simulink model "modules"  (R2017a)
settings: Solver=ode4  StartTime=0.0  StopTime=time_stop  FixedStep=time_step  RelTol=1e-3
values from neighbouring files (symbols this model uses):
  psi = state(3)    [PSVobstacleShip_class.m]    (also in PSVvessel_class.m = obj.eta(3); PsiReferenceModel_class.m = obj.desired_psi_vector; SBMPC_PSVvessel_class.m = obj.eta(3))
undefined symbols (not defined in the file or in its folder): beta, Delta_guidance, Delta_matrix, eta_initial, initial_desired_psi_vector, initial_desired_u_vector, initial_next_waypoint_indexes, initial_obstacle_ship_states, initial_obstacle_ship_states_dot, initial_reference_psi_vector, initial_reference_u_vector, initial_SBMPC_desired_psi_vector, initial_SBMPC_desired_u_vector, initial_SBMPC_next_waypoint_indexes, initial_SBMPC_obstacle_ship_states, initial_SBMPC_obstacle_ship_states_dot, initial_SBMPC_reference_psi_vector, initial_SBMPC_reference_u_vector, initial_SBMPC_x_d_psi_matrix, initial_SBMPC_x_d_u_matrix, initial_state, initial_x_d_psi_matrix, initial_x_d_u_matrix, K_sway, K_yaw, Kp_feedback_linearization, kp_heading, Nmax, nu_initial, num_obs_ship_waypoints, num_prediction_time_steps, number_of_control_behaviors, number_of_obstacle_ships, number_of_SBMPC_obstacle_ships, obs_speed_between_waypoints, obstacle_waypoint_matrix, Omega_matrix, own_ship_reference_psi_init, own_ship_reference_speed, Psi_init, radius_of_acceptance, SBMPC_obs_speed_between_waypoints, SBMPC_obstacle_waypoint_matrix, seconds_between_prediction, state_vector_init, T, T_k_surge, T_k_sway, T_k_yaw, T_s, T_waypoints, time_step, tsamp, U, U_init, V_init, waypoints_obstacle_ships, waypoints_own_ship, Xmax, Ymax
(part 1 of 5)
settings Model: TunableVars=eta_initial,nu_initial,waypoints_own_ship,waypoints_own_ship_straight_path  TunableVarsStorageClass=Auto,Auto,Auto,Auto  TunableVarsTypeQualifier=,,,  Creator=krikjers  LastModifiedBy=Kristian
settings DataIOCC: SaveFormat=Structure
settings RTWCC: SystemTargetFile=grtfmi.tlc  GenerateMakefile=off  TemplateMakefile=none  Description=FMU based on GRT (Functional Mock-up Unit)  RetainRTWFile=on
settings STFCustomTargetCC: TargetLangStandard=C99 (ISO)  CombineOutputUpdateFcns=on  MultiInstanceERTCode=on  CodeInterfacePackaging=Reusable function  GRTInterface=off  GenerateAllocFcn=on  SystemTargetFile=grtfmi.tlc
settings GRTTargetCC: ParMdlRefBuildCompliant=off  CompOptLevelCompliant=off  ConcurrentExecutionCompliant=off  MatFileLogging=off  MultiInstanceERTCode=on  CodeInterfacePackaging=Reusable function  CPPClassGenCompliant=off  GenerateAllocFcn=on  UseToolchainInfoCompliant=off

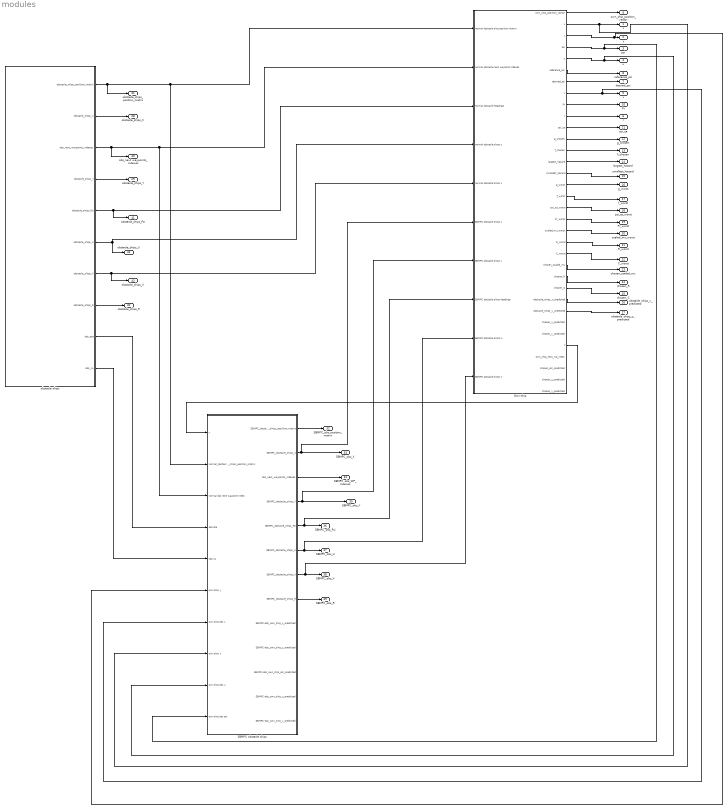
== system modules ==
  Own-ship : Subsystem
  SBMPC obstacle ships : Subsystem
  obstacle ships : Subsystem
  x : Outport
  y : Outport  Port=2
  psi : Outport  Port=3
  u : Outport  Port=4
  v : Outport  Port=5
  r : Outport  Port=6
  desired_psi : Outport  Port=7
  reference_psi : Outport  Port=8
  "own_ship_position_vector " : Outport  Port=9
  Pr : Outport  Port=10
  "psi_ca " : Outport  Port=11
  "g_chosen " : Outport  Port=12  SampleTime=time_step
  f_chosen : Outport  Port=13  SampleTime=time_step
  largest_hazard : Outport  Port=14  SampleTime=time_step
  smallest_hazard : Outport  Port=15  SampleTime=time_step
  "g_worst " : Outport  Port=16  SampleTime=time_step
  f_worst : Outport  Port=17  SampleTime=time_step
  psi_ca_worst : Outport  Port=18  SampleTime=time_step
  Pr_worst : Outport  Port=19  SampleTime=time_step
  scaled_mu_worst : Outport  Port=20  SampleTime=time_step
  R_worst : Outport  Port=21  SampleTime=time_step
  C_worst : Outport  Port=22  SampleTime=time_step
  chosen_scaled_mu : Outport  Port=23  SampleTime=time_step
  chosen_R : Outport  Port=24  SampleTime=time_step
  chosen_C : Outport  Port=25  SampleTime=time_step
  obstacle_ships_x_predicted : Outport  Port=26  SampleTime=time_step
  "obstacle_ships_y_predicted " : Outport  Port=27  SampleTime=time_step
  obstacle_ships_X : Outport  Port=28
  obstacle_ships_Y : Outport  Port=29
  obstacle_ships_R : Outport  Port=30
  "obstacle_ships_position_matrix " : Outport  Port=31
  "SBMPC_obs_position_matrix " : Outport  Port=32
  SBMPC_obs_X : Outport  Port=33
  SBMPC_obs_WP_indexes : Outport  Port=34
  SBMPC_obs_Y : Outport  Port=35
  SBMPC_obs_Psi : Outport  Port=36
  SBMPC_obs_U : Outport  Port=37
  SBMPC_obs_V : Outport  Port=38
  SBMPC_obs_R : Outport  Port=39
  obs_next_waypoints_indexes : Outport  Port=40
  obstacle_ships_Psi : Outport  Port=41
  obstacle_ships_U : Outport  Port=42
  obstacle_ships_V : Outport  Port=43
  wires:
  obstacle ships/2(obstacle_ships_X) -> obstacle_ships_X/1
  obstacle ships/4(obstacle_ships_Y) -> obstacle_ships_Y/1
  obstacle ships/5(obstacle_ships_Psi) -> obstacle_ships_Psi/1, Own-ship/3(normal obstacle headings)
  obstacle ships/6(obstacle_ships_U) -> obstacle_ships_U/1, Own-ship/4(normal obstacle ships u)
  obstacle ships/7(obstacle_ships_V) -> obstacle_ships_V/1, Own-ship/5(normal obstacle ships v)
  obstacle ships/8(obstacle_ships_R) -> obstacle_ships_R/1
  obstacle ships/3(obs_next_waypoints_indexes) -> obs_next_waypoints_indexes/1, Own-ship/2(normal obstacle next waypoint indexes), SBMPC obstacle ships/3(normal obs next waypoint index)
  Own-ship/1("own_ship_position_vector ") -> "own_ship_position_vector "/1
  Own-ship/2(x) -> SBMPC obstacle ships/8("own ship  x "), x/1
  Own-ship/6(reference_psi) -> reference_psi/1
  Own-ship/7(desired_psi) -> desired_psi/1
  Own-ship/9(Pr) -> Pr/1
  Own-ship/10(r) -> r/1
  Own-ship/11("psi_ca ") -> "psi_ca "/1
  Own-ship/12("g_chosen ") -> "g_chosen "/1
  Own-ship/13(f_chosen) -> f_chosen/1
  Own-ship/14(largest_hazard) -> largest_hazard/1
  Own-ship/15(smallest_hazard) -> smallest_hazard/1
  Own-ship/16("g_worst ") -> "g_worst "/1
  Own-ship/17(f_worst) -> f_worst/1
  Own-ship/18(psi_ca_worst) -> psi_ca_worst/1
  Own-ship/19(Pr_worst) -> Pr_worst/1
  Own-ship/20(scaled_mu_worst) -> scaled_mu_worst/1
  Own-ship/21(R_worst) -> R_worst/1
  Own-ship/22(C_worst) -> C_worst/1
  Own-ship/23(chosen_scaled_mu) -> chosen_scaled_mu/1
  Own-ship/24(chosen_R) -> chosen_R/1
  Own-ship/25(chosen_C) -> chosen_C/1
  Own-ship/26(obstacle_ships_x_predicted) -> obstacle_ships_x_predicted/1
  Own-ship/27("obstacle_ships_y_predicted ") -> "obstacle_ships_y_predicted "/1
  SBMPC obstacle ships/7(SBMPC_obstacle_ships_V) -> SBMPC_obs_V/1, Own-ship/10("SBMPC obstacle ships V ")
  SBMPC obstacle ships/6(SBMPC_obstacle_ships_U) -> Own-ship/9("SBMPC obstacle ships U "), SBMPC_obs_U/1
  SBMPC obstacle ships/5(SBMPC_obstacle_ships_Psi) -> Own-ship/8("SBMPC obstacle ships headings "), SBMPC_obs_Psi/1
  SBMPC obstacle ships/8(SBMPC_obstacle_ships_R) -> SBMPC_obs_R/1
  SBMPC obstacle ships/4(SBMPC_obstacle_ships_Y) -> Own-ship/7("SBMPC obstacle ships y "), SBMPC_obs_Y/1
  SBMPC obstacle ships/3(obs_next_waypoints_indexes) -> SBMPC_obs_WP_indexes/1
  SBMPC obstacle ships/2(SBMPC_obstacle_ships_X) -> Own-ship/6("SBMPC obstacle ships x "), SBMPC_obs_X/1
  SBMPC obstacle ships/1("SBMPC_obstacle_ships_positiion_matrix ") -> "SBMPC_obs_position_matrix "/1
  Own-ship/30(t) -> SBMPC obstacle ships/1(t)
  obstacle ships/9(obs_eta) -> SBMPC obstacle ships/4(obs eta)
  obstacle ships/10(obs_nu) -> SBMPC obstacle ships/5(obs nu)
  obstacle ships/1("obstacle_ships_positiion_matrix ") -> "obstacle_ships_position_matrix "/1, SBMPC obstacle ships/2(normal_obstacle_ships_position_matrix), Own-ship/1("normal obstacle ship position matrix ")
  Own-ship/5(u) -> SBMPC obstacle ships/9("own ship obs u "), u/1
  Own-ship/8(v) -> SBMPC obstacle ships/7("own ship obs v "), v/1
  Own-ship/4(psi) -> SBMPC obstacle ships/10("own ship obs psi "), psi/1
  Own-ship/3(y) -> SBMPC obstacle ships/6("own ship  y "), y/1

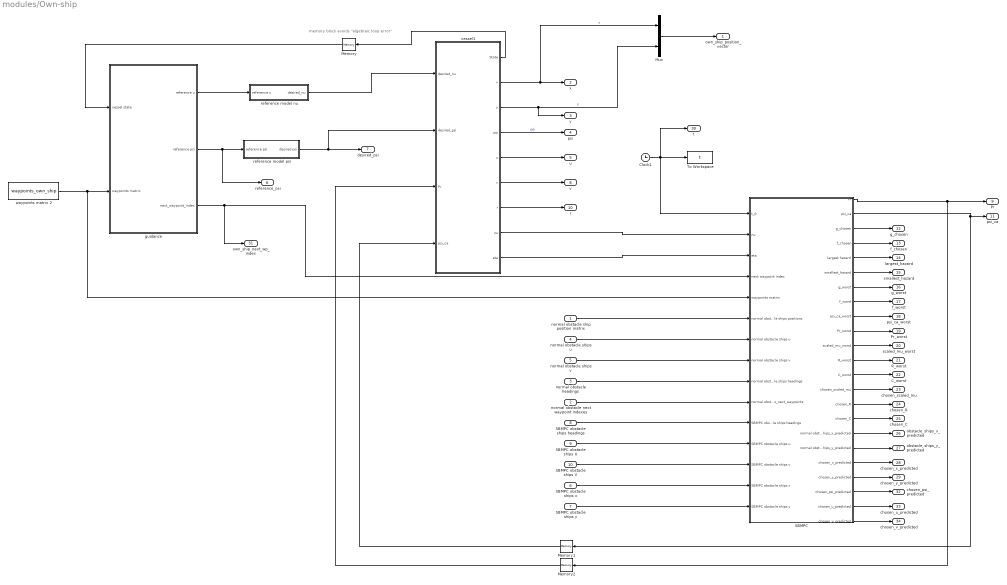
== system modules/Own-ship ==
  note: memory block avoids "algebraic loop error"
  "normal obstacle ship position matrix " : Inport
  normal obstacle next waypoint indexes : Inport  Port=2
  normal obstacle headings : Inport  Port=3
  normal obstacle ships u : Inport  Port=4
  normal obstacle ships v : Inport  Port=5
  "SBMPC obstacle ships x " : Inport  Port=6
  "SBMPC obstacle ships y " : Inport  Port=7
  "SBMPC obstacle ships headings " : Inport  Port=8
  "SBMPC obstacle ships U " : Inport  Port=9
  "SBMPC obstacle ships V " : Inport  Port=10
  Clock1 : Clock
  Memory : Memory  X0=initial_state  InheritSampleTime=on
  Memory1 : Memory  InheritSampleTime=on
  Memory2 : Memory  InheritSampleTime=on
  Mux : Mux  Inputs=2
  "SBMPC " : Subsystem
  To Workspace : ToWorkspace  VariableName=t  SampleTime=tsamp
  guidance : Subsystem
  reference model nu : Subsystem
  reference model psi : Subsystem
  vessel1 : Subsystem
  waypoints matrix 2 : Constant  Value=waypoints_own_ship  VectorParams1D=off  SampleTime=time_step
  "own_ship_position_vector " : Outport
  x : Outport  Port=2
  y : Outport  Port=3
  psi : Outport  Port=4
  u : Outport  Port=5
  reference_psi : Outport  Port=6
  desired_psi : Outport  Port=7
  v : Outport  Port=8
  Pr : Outport  Port=9
  r : Outport  Port=10
  "psi_ca " : Outport  Port=11
  "g_chosen " : Outport  Port=12  SampleTime=time_step
  f_chosen : Outport  Port=13  SampleTime=time_step
  largest_hazard : Outport  Port=14  SampleTime=time_step
  smallest_hazard : Outport  Port=15  SampleTime=time_step
  "g_worst " : Outport  Port=16  SampleTime=time_step
  f_worst : Outport  Port=17  SampleTime=time_step
  psi_ca_worst : Outport  Port=18  SampleTime=time_step
  Pr_worst : Outport  Port=19  SampleTime=time_step
  scaled_mu_worst : Outport  Port=20  SampleTime=time_step
  R_worst : Outport  Port=21  SampleTime=time_step
  C_worst : Outport  Port=22  SampleTime=time_step
  chosen_scaled_mu : Outport  Port=23  SampleTime=time_step
  chosen_R : Outport  Port=24  SampleTime=time_step
  chosen_C : Outport  Port=25  SampleTime=time_step
  obstacle_ships_x_predicted : Outport  Port=26  SampleTime=time_step
  "obstacle_ships_y_predicted " : Outport  Port=27  SampleTime=time_step
  chosen_x_predicted : Outport  Port=28  SampleTime=time_step
  chosen_y_predicted : Outport  Port=29  SampleTime=time_step
  t : Outport  Port=30
  own_ship_next_wp_index : Outport  Port=31
  chosen_psi_predicted : Outport  Port=32  SampleTime=time_step
  "chosen_u_predicted " : Outport  Port=33  SampleTime=time_step
  chosen_v_predicted : Outport  Port=34  SampleTime=time_step
  wires:
  vessel1/5(u) -> u/1
  vessel1/6(v) -> v/1
  vessel1/3(y) -> y/1, Mux/2  "y"
  Memory2/1 -> vessel1/3(Pr)
  Memory/1 -> guidance/1(vessel state)
  vessel1/9(eta) -> "SBMPC "/3(eta)
  waypoints matrix 2/1 -> "SBMPC "/5("waypoints matrix "), guidance/2("waypoints matrix ")
  "SBMPC "/4(f_chosen) -> f_chosen/1
  "SBMPC "/6(smallest_hazard) -> smallest_hazard/1
  "SBMPC "/7("g_worst ") -> "g_worst "/1
  "SBMPC "/8(f_worst) -> f_worst/1
  "SBMPC "/9(psi_ca_worst) -> psi_ca_worst/1
  guidance/2("reference psi ") -> reference_psi/1, reference model psi/1(reference psi)
  "SBMPC "/2(psi_ca) -> Memory1/1, "psi_ca "/1
  guidance/3(next_waypoint_index) -> own_ship_next_wp_index/1, "SBMPC "/4(next waypoint index)
  reference model psi/1(desired psi) -> desired_psi/1, vessel1/2("desired_psi ")
  vessel1/4(psi) -> psi/1  "psi"
  Memory1/1 -> vessel1/4(psi_ca)
  "SBMPC "/3("g_chosen ") -> "g_chosen "/1
  guidance/1(reference u) -> reference model nu/1(reference u)
  Mux/1 -> "own_ship_position_vector "/1
  "SBMPC "/5(largest hazard) -> largest_hazard/1
  vessel1/1("State ") -> Memory/1
  reference model nu/1(desired_nu) -> vessel1/1(desired_nu)
  vessel1/2(x) -> x/1, Mux/1  "x"
  Clock1/1 -> t/1, "SBMPC "/1(t_0), To Workspace/1
  vessel1/7(r) -> r/1
  vessel1/8(nu) -> "SBMPC "/2(nu)
  "SBMPC "/1(Pr) -> Memory2/1, Pr/1
  "SBMPC "/10(Pr_worst) -> Pr_worst/1
  "SBMPC "/18("normal obstacle_ships_y_predicted ") -> "obstacle_ships_y_predicted "/1
  "SBMPC "/13(C_worst) -> C_worst/1
  "SBMPC "/17(normal obstacle_ships_x_predicted) -> obstacle_ships_x_predicted/1
  "SBMPC "/12(R_worst) -> R_worst/1
  "SBMPC "/14(chosen_scaled_mu) -> chosen_scaled_mu/1
  "SBMPC "/15(chosen_R) -> chosen_R/1
  "SBMPC "/11(scaled_mu_worst) -> scaled_mu_worst/1
  "SBMPC "/16(chosen_C) -> chosen_C/1
  "normal obstacle ship position matrix "/1 -> "SBMPC "/6(normal obstacle ships positions)
  normal obstacle ships u/1 -> "SBMPC "/7(normal obstacle ships u)
  normal obstacle ships v/1 -> "SBMPC "/8(normal obstacle ships v)
  normal obstacle next waypoint indexes/1 -> "SBMPC "/10(normal obstacle_ships_next_waypoints)
  normal obstacle headings/1 -> "SBMPC "/9(normal obstacle ships headings)
  "SBMPC obstacle ships headings "/1 -> "SBMPC "/11(SBMPC obstacle ships headings)
  "SBMPC obstacle ships U "/1 -> "SBMPC "/12(SBMPC obstacle ships u)
  "SBMPC obstacle ships V "/1 -> "SBMPC "/13(SBMPC obstacle ships v)
  "SBMPC "/19(chosen_x_predicted) -> chosen_x_predicted/1
  "SBMPC "/20(chosen_y_predicted) -> chosen_y_predicted/1
  "SBMPC obstacle ships x "/1 -> "SBMPC "/14("SBMPC obstacle ships x ")
  "SBMPC obstacle ships y "/1 -> "SBMPC "/15("SBMPC obstacle ships y ")
  "SBMPC "/21(chosen_psi_predicted) -> chosen_psi_predicted/1
  "SBMPC "/22(chosen_u_predicted) -> "chosen_u_predicted "/1
  "SBMPC "/23(chosen_v_predicted) -> chosen_v_predicted/1

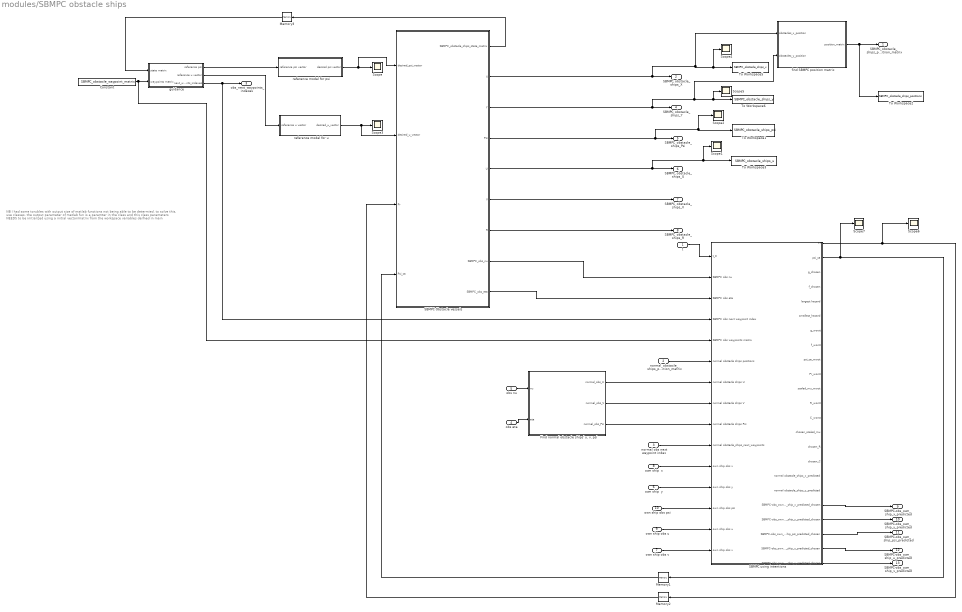
== system modules/SBMPC obstacle ships ==
  note: NB I had some torubles with output size of matlab functions not being able to be determied.
      | to solve this, use classes. the output parameter of matlab fun is a paramter in the class and this
      | class parameters NEEDS to be initialized using a initial vector/matrix from the workspace variables
      | deifned in main
  t : Inport
  normal_obstacle_ships_position_matrix : Inport  Port=2
  normal obs next waypoint index : Inport  Port=3
  obs eta : Inport  Port=4
  obs nu : Inport  Port=5
  "own ship  y " : Inport  Port=6
  "own ship obs v " : Inport  Port=7
  "own ship  x " : Inport  Port=8
  "own ship obs u " : Inport  Port=9
  "own ship obs psi " : Inport  Port=10
  Constant : Constant  Value=SBMPC_obstacle_waypoint_matrix  VectorParams1D=off
  "Find normal obstacle ships' u, v, psi" : MATLAB Function  TreatAsAtomicUnit=on
  Memory1 : Memory  InheritSampleTime=on
  Memory2 : Memory  InheritSampleTime=on
  Memory3 : Memory
  SBMPC Obstacle vessels : MATLAB Function  TreatAsAtomicUnit=on
  "SBMPC using intentions " : Subsystem
  Scope{,1..7} (8 alike) : Scope
  To Workspace1 : ToWorkspace  VariableName=SBMPC_obstacle_ships_psi  SampleTime=tsamp
      settings: Save2DSignal=2-D array (concatenate along first dimension)
  To Workspace2 : ToWorkspace  VariableName=SBMPC_obstacle_ships_positions  SampleTime=tsamp
  To Workspace3 : ToWorkspace  VariableName=SBMPC_obstacle_ships_u  SampleTime=tsamp
      settings: Save2DSignal=2-D array (concatenate along first dimension)
  To Workspace5 : ToWorkspace  VariableName=SBMPC_obstacle_ships_x  SampleTime=tsamp
      settings: Save2DSignal=2-D array (concatenate along first dimension)
  To Workspace6 : ToWorkspace  VariableName=SBMPC_obstacle_ships_y  SampleTime=tsamp
      settings: Save2DSignal=2-D array (concatenate along first dimension)
  find SBMPC position matrix : MATLAB Function  TreatAsAtomicUnit=on
  "guidance " : Subsystem
  reference model for psi : Subsystem
  reference model for u : Subsystem
  "SBMPC_obstacle_ships_positiion_matrix " : Outport
  SBMPC_obstacle_ships_X : Outport  Port=2
  obs_next_waypoints_indexes : Outport  Port=3
  SBMPC_obstacle_ships_Y : Outport  Port=4
  SBMPC_obstacle_ships_Psi : Outport  Port=5
  SBMPC_obstacle_ships_U : Outport  Port=6
  SBMPC_obstacle_ships_V : Outport  Port=7
  SBMPC_obstacle_ships_R : Outport  Port=8
  SBMPC-obs_own_ship_x_predicted : Outport  Port=9  SampleTime=time_step
  SBMPC-obs_own_ship_y_predicted : Outport  Port=10  SampleTime=time_step
  SBMPC-obs_own_ship_psi_predicted : Outport  Port=11  SampleTime=time_step
  SBMPC-obs_own_ship_u_predicted : Outport  Port=12  SampleTime=time_step
  SBMPC-obs_own_ship_v_predicted : Outport  Port=13  SampleTime=time_step
  wires:
  SBMPC Obstacle vessels/1(SBMPC_obstacle_ships_state_matrix) -> Memory3/1
  SBMPC Obstacle vessels/6(V) -> SBMPC_obstacle_ships_V/1
  reference model for u/1(desired_u_vector) -> SBMPC Obstacle vessels/2(desired_u_vector), Scope3/1
  "guidance "/1("reference psi ") -> reference model for psi/1(reference psi vector)
  SBMPC Obstacle vessels/3(Y) -> SBMPC_obstacle_ships_Y/1, find SBMPC position matrix/2(obstacles_y_position), Scope5/1, To Workspace6/1
  Constant/1 -> "SBMPC using intentions "/5("SBMPC obs waypoints matrix "), "guidance "/2("waypoints matrix ")
  SBMPC Obstacle vessels/2(X) -> SBMPC_obstacle_ships_X/1, find SBMPC position matrix/1(obstacles_x_position), Scope4/1, To Workspace5/1
  reference model for psi/1("desired psi vector ") -> SBMPC Obstacle vessels/1(desired_psi_vector), Scope/1
  find SBMPC position matrix/1(position_matrix) -> To Workspace2/1, "SBMPC_obstacle_ships_positiion_matrix "/1
  Memory3/1 -> "guidance "/1(state matrix)
  "guidance "/2(reference u vector) -> reference model for u/1("reference u vector ")
  SBMPC Obstacle vessels/4(Psi) -> SBMPC_obstacle_ships_Psi/1, Scope2/1, To Workspace1/1
  SBMPC Obstacle vessels/7(R) -> SBMPC_obstacle_ships_R/1
  "SBMPC using intentions "/2(psi_ca) -> Scope7/1, Memory1/1
  t/1 -> "SBMPC using intentions "/1(t_0)
  SBMPC Obstacle vessels/8(SBMPC_obs_nu) -> "SBMPC using intentions "/2(SBMPC obs nu)
  SBMPC Obstacle vessels/9(SBMPC_obs_eta) -> "SBMPC using intentions "/3(SBMPC obs eta)
  "guidance "/3("next_waypoints_indexes ") -> "SBMPC using intentions "/4(SBMPC obs next waypoint index), obs_next_waypoints_indexes/1
  SBMPC Obstacle vessels/5(U) -> SBMPC_obstacle_ships_U/1, Scope1/1, To Workspace3/1
  obs eta/1 -> "Find normal obstacle ships' u, v, psi"/2(eta)
  normal obs next waypoint index/1 -> "SBMPC using intentions "/10(normal obstacle_ships_next_waypoints)
  normal_obstacle_ships_position_matrix/1 -> "SBMPC using intentions "/6(normal obstacle ships positions)
  obs nu/1 -> "Find normal obstacle ships' u, v, psi"/1(nu)
  "Find normal obstacle ships' u, v, psi"/1(normal_obs_U) -> "SBMPC using intentions "/7(normal obstacle ships U)
  "Find normal obstacle ships' u, v, psi"/2(normal_obs_V) -> "SBMPC using intentions "/8(normal obstacle ships V)
  "Find normal obstacle ships' u, v, psi"/3(normal_obs_Psi) -> "SBMPC using intentions "/9(normal obstacle ships Psi)
  "own ship obs u "/1 -> "SBMPC using intentions "/14("own ship obs u ")
  "own ship obs v "/1 -> "SBMPC using intentions "/15("own ship obs v ")
  "own ship obs psi "/1 -> "SBMPC using intentions "/13("own ship obs psi ")
  "own ship  x "/1 -> "SBMPC using intentions "/11("own ship obs x ")
  "own ship  y "/1 -> "SBMPC using intentions "/12("own ship obs y ")
  "SBMPC using intentions "/19(SBMPC-obs_own_ship_x_predicted_chosen) -> SBMPC-obs_own_ship_x_predicted/1
  "SBMPC using intentions "/20(SBMPC-obs_own_ship_y_predicted_chosen) -> SBMPC-obs_own_ship_y_predicted/1
  "SBMPC using intentions "/21(SBMPC-obs_own_ship_psi_predicted_chosen) -> SBMPC-obs_own_ship_psi_predicted/1
  "SBMPC using intentions "/22(SBMPC-obs_own_ship_u_predicted_chosen) -> SBMPC-obs_own_ship_u_predicted/1
  "SBMPC using intentions "/23(SBMPC-obs_own_ship_v_predicted_chosen) -> SBMPC-obs_own_ship_v_predicted/1
  "SBMPC using intentions "/1(Pr) -> Scope6/1, Memory2/1
  Memory2/1 -> SBMPC Obstacle vessels/3(Pr)
  Memory1/1 -> SBMPC Obstacle vessels/4(Psi_ca)

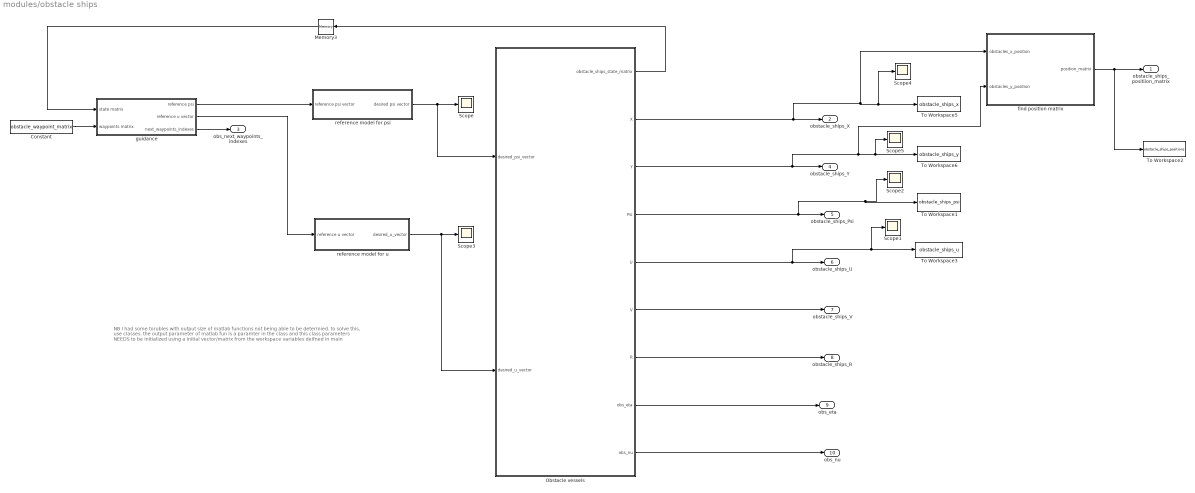
== system modules/obstacle ships ==
  note: NB I had some torubles with output size of matlab functions not being able to be determied.
      | to solve this, use classes. the output parameter of matlab fun is a paramter in the class and this
      | class parameters NEEDS to be initialized using a initial vector/matrix from the workspace variables
      | deifned in main
  Constant : Constant  Value=obstacle_waypoint_matrix  VectorParams1D=off
  Memory3 : Memory
  Obstacle vessels : MATLAB Function  TreatAsAtomicUnit=on
  Scope{,1..5} (6 alike) : Scope
  To Workspace1 : ToWorkspace  VariableName=obstacle_ships_psi  SampleTime=tsamp
      settings: Save2DSignal=2-D array (concatenate along first dimension)
  To Workspace2 : ToWorkspace  VariableName=obstacle_ships_positions  SampleTime=tsamp
  To Workspace3 : ToWorkspace  VariableName=obstacle_ships_u  SampleTime=tsamp
      settings: Save2DSignal=2-D array (concatenate along first dimension)
  To Workspace5 : ToWorkspace  VariableName=obstacle_ships_x  SampleTime=tsamp
      settings: Save2DSignal=2-D array (concatenate along first dimension)
  To Workspace6 : ToWorkspace  VariableName=obstacle_ships_y  SampleTime=tsamp
      settings: Save2DSignal=2-D array (concatenate along first dimension)
  find position matrix : MATLAB Function  TreatAsAtomicUnit=on
  "guidance " : Subsystem
  reference model for psi : Subsystem
  reference model for u : Subsystem
  "obstacle_ships_positiion_matrix " : Outport
  obstacle_ships_X : Outport  Port=2
  obs_next_waypoints_indexes : Outport  Port=3
  obstacle_ships_Y : Outport  Port=4
  obstacle_ships_Psi : Outport  Port=5
  obstacle_ships_U : Outport  Port=6
  obstacle_ships_V : Outport  Port=7
  obstacle_ships_R : Outport  Port=8
  obs_eta : Outport  Port=9
  obs_nu : Outport  Port=10
  wires:
  Obstacle vessels/1(obstacle_ships_state_matrix) -> Memory3/1
  Obstacle vessels/6(V) -> obstacle_ships_V/1
  reference model for u/1(desired_u_vector) -> Obstacle vessels/2(desired_u_vector), Scope3/1
  "guidance "/1("reference psi ") -> reference model for psi/1(reference psi vector)
  Obstacle vessels/5(U) -> obstacle_ships_U/1, Scope1/1, To Workspace3/1
  Constant/1 -> "guidance "/2("waypoints matrix ")
  "guidance "/3("next_waypoints_indexes ") -> obs_next_waypoints_indexes/1
  Obstacle vessels/2(X) -> obstacle_ships_X/1, find position matrix/1(obstacles_x_position), Scope4/1, To Workspace5/1
  reference model for psi/1("desired psi vector ") -> Obstacle vessels/1(desired_psi_vector), Scope/1
  find position matrix/1(position_matrix) -> To Workspace2/1, "obstacle_ships_positiion_matrix "/1
  Memory3/1 -> "guidance "/1(state matrix)
  "guidance "/2(reference u vector) -> reference model for u/1("reference u vector ")
  Obstacle vessels/4(Psi) -> obstacle_ships_Psi/1, Scope2/1, To Workspace1/1
  Obstacle vessels/7(R) -> obstacle_ships_R/1
  Obstacle vessels/3(Y) -> obstacle_ships_Y/1, find position matrix/2(obstacles_y_position), Scope5/1, To Workspace6/1
  Obstacle vessels/8(obs_eta) -> obs_eta/1
  Obstacle vessels/9(obs_nu) -> obs_nu/1

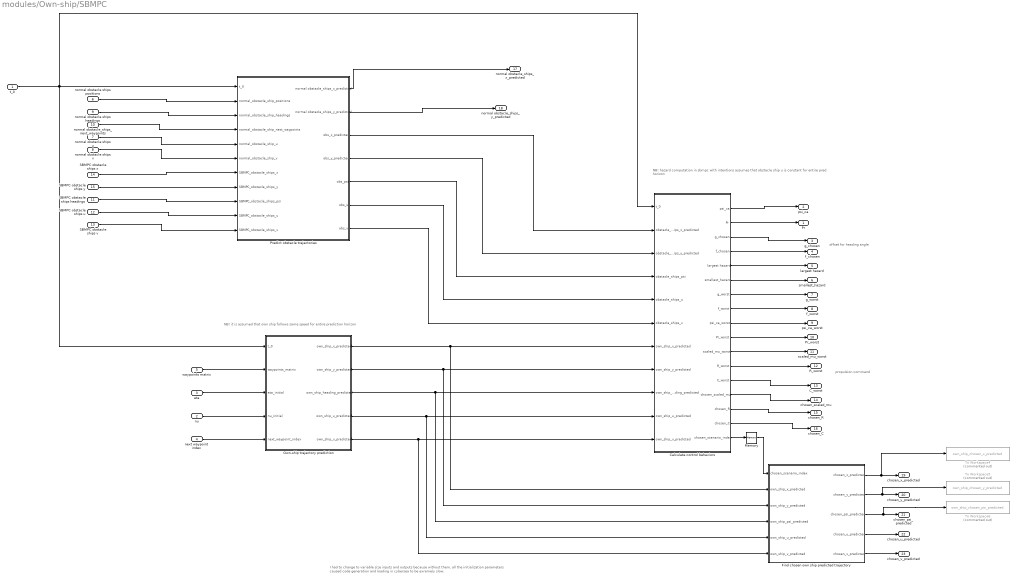
== system modules/Own-ship/SBMPC  ==
  note: NB! hazard computation in sbmpc with intentions assumes that obstacle ship u is constant for entire pred horizon
  note: NB! it is assumed that own ship follows same speed for entire prediction horizon
  note: I had to change to variable size inputs and outputs because without them, all the initialization parameters caused
      | code generation and loading in cybersea to be exremely slow.
  note: propulsion command
  note: offset for heading angle
  t_0 : Inport
  nu : Inport  Port=2
  eta : Inport  Port=3
  next waypoint index : Inport  Port=4
  "waypoints matrix " : Inport  Port=5
  normal obstacle ships positions : Inport  Port=6
  normal obstacle ships u : Inport  Port=7
  normal obstacle ships v : Inport  Port=8
  normal obstacle ships headings : Inport  Port=9
  normal obstacle_ships_next_waypoints : Inport  Port=10
  SBMPC obstacle ships headings : Inport  Port=11
  SBMPC obstacle ships u : Inport  Port=12
  SBMPC obstacle ships v : Inport  Port=13
  "SBMPC obstacle ships x " : Inport  Port=14
  "SBMPC obstacle ships y " : Inport  Port=15
  Calculate control behaviors : Subsystem
  Find chosen own ship predicted trajectory : MATLAB Function  TreatAsAtomicUnit=on
  Memory : Memory  X0=7
  Own-ship trajectory prediction : Subsystem
  Predict obstacle trajectories : Subsystem
  To Workspace4 : ToWorkspace  Commented=on  VariableName=own_ship_chosen_x_predicted  SaveFormat=Structure With Time  SampleTime=tsamp
      settings: Save2DSignal=2-D array (concatenate along first dimension)
  To Workspace5 : ToWorkspace  Commented=on  VariableName=own_ship_chosen_y_predicted  SaveFormat=Structure With Time  SampleTime=tsamp
      settings: Save2DSignal=2-D array (concatenate along first dimension)
  To Workspace6 : ToWorkspace  Commented=on  VariableName=own_ship_chosen_psi_predicted  SaveFormat=Structure With Time  SampleTime=tsamp
      settings: Save2DSignal=2-D array (concatenate along first dimension)
  Pr : Outport
  psi_ca : Outport  Port=2
  "g_chosen " : Outport  Port=3  SampleTime=time_step
  f_chosen : Outport  Port=4  SampleTime=time_step
  largest hazard : Outport  Port=5  SampleTime=time_step
  smallest_hazard : Outport  Port=6  SampleTime=time_step
  "g_worst " : Outport  Port=7  SampleTime=time_step
  f_worst : Outport  Port=8  SampleTime=time_step
  psi_ca_worst : Outport  Port=9  SampleTime=time_step
  Pr_worst : Outport  Port=10  SampleTime=time_step
  scaled_mu_worst : Outport  Port=11  SampleTime=time_step
  R_worst : Outport  Port=12  SampleTime=time_step
  C_worst : Outport  Port=13  SampleTime=time_step
  chosen_scaled_mu : Outport  Port=14  SampleTime=time_step
  chosen_R : Outport  Port=15  SampleTime=time_step
  chosen_C : Outport  Port=16  SampleTime=time_step
  normal obstacle_ships_x_predicted : Outport  Port=17  SampleTime=time_step
  "normal obstacle_ships_y_predicted " : Outport  Port=18  SampleTime=time_step
  chosen_x_predicted : Outport  Port=19  SampleTime=time_step
  chosen_y_predicted : Outport  Port=20  SampleTime=time_step
  chosen_psi_predicted : Outport  Port=21  SampleTime=time_step
  chosen_u_predicted : Outport  Port=22  SampleTime=time_step
  chosen_v_predicted : Outport  Port=23  SampleTime=time_step
  wires:
  "waypoints matrix "/1 -> Own-ship trajectory prediction/2(waypoints_matrix)
  eta/1 -> Own-ship trajectory prediction/3("eta_initial ")
  nu/1 -> Own-ship trajectory prediction/4(nu_initial)
  next waypoint index/1 -> Own-ship trajectory prediction/5(next_waypoint_index)
  t_0/1 -> Own-ship trajectory prediction/1(t_0), Predict obstacle trajectories/1(t_0), Calculate control behaviors/1(t_0)
  Own-ship trajectory prediction/1(own_ship_x_predicted) -> Find chosen own ship predicted trajectory/2(own_ship_x_predicted), Calculate control behaviors/7(own_ship_x_predicted)
  Own-ship trajectory prediction/4(own_ship_u_predicted) -> Find chosen own ship predicted trajectory/5(own_ship_u_predicted), Calculate control behaviors/10(own_ship_u_predicted)
  Own-ship trajectory prediction/5("own_ship_v_predicted ") -> Find chosen own ship predicted trajectory/6(own_ship_v_predicted), Calculate control behaviors/11("own_ship_v_predicted ")
  Own-ship trajectory prediction/3(own_ship_heading_predicted) -> Find chosen own ship predicted trajectory/4(own_ship_psi_predicted), Calculate control behaviors/9("own_ship_heading_predicted ")
  Calculate control behaviors/2(Pr) -> Pr/1
  Calculate control behaviors/1(psi_ca) -> psi_ca/1
  Calculate control behaviors/16(chosen_C) -> chosen_C/1
  Calculate control behaviors/15(chosen_R) -> chosen_R/1
  Calculate control behaviors/14(chosen_scaled_mu) -> chosen_scaled_mu/1
  Calculate control behaviors/13(C_worst) -> C_worst/1
  Calculate control behaviors/12(R_worst) -> R_worst/1
  Calculate control behaviors/11(scaled_mu_worst) -> scaled_mu_worst/1
  Calculate control behaviors/10(Pr_worst) -> Pr_worst/1
  Calculate control behaviors/9(psi_ca_worst) -> psi_ca_worst/1
  Calculate control behaviors/8(f_worst) -> f_worst/1
  Calculate control behaviors/7("g_worst ") -> "g_worst "/1
  Calculate control behaviors/6(smallest_hazard) -> smallest_hazard/1
  Calculate control behaviors/5(largest hazard) -> largest hazard/1
  Calculate control behaviors/4(f_chosen) -> f_chosen/1
  Calculate control behaviors/3("g_chosen ") -> "g_chosen "/1
  Find chosen own ship predicted trajectory/1(chosen_x_predicted) -> To Workspace4/1, chosen_x_predicted/1
  Find chosen own ship predicted trajectory/2(chosen_y_predicted) -> To Workspace5/1, chosen_y_predicted/1
  Calculate control behaviors/17("chosen_scenario_index ") -> Memory/1
  Memory/1 -> Find chosen own ship predicted trajectory/1(chosen_scenario_index)
  Find chosen own ship predicted trajectory/4(chosen_u_predicted) -> chosen_u_predicted/1
  Find chosen own ship predicted trajectory/5(chosen_v_predicted) -> chosen_v_predicted/1
  Own-ship trajectory prediction/2(own_ship_y_predicted) -> Find chosen own ship predicted trajectory/3(own_ship_y_predicted), Calculate control behaviors/8(own_ship_y_predicted)
  Find chosen own ship predicted trajectory/3(chosen_psi_predicted) -> To Workspace6/1, chosen_psi_predicted/1
  normal obstacle ships positions/1 -> Predict obstacle trajectories/2(normal_obstacle_ship_positions)
  normal obstacle ships headings/1 -> Predict obstacle trajectories/3(normal_obstacle_ship_headings)
  normal obstacle_ships_next_waypoints/1 -> Predict obstacle trajectories/4(normal_obstacle_ship_next_waypoints)
  normal obstacle ships u/1 -> Predict obstacle trajectories/5(normal_obstacle_ship_u)
  normal obstacle ships v/1 -> Predict obstacle trajectories/6(normal_obstacle_ship_v)
  "SBMPC obstacle ships x "/1 -> Predict obstacle trajectories/7(SBMPC_obstacle_ships_x)
  "SBMPC obstacle ships y "/1 -> Predict obstacle trajectories/8(SBMPC_obstacle_ships_y)
  SBMPC obstacle ships headings/1 -> Predict obstacle trajectories/9(SBMPC_obstacle_ships_psi)
  SBMPC obstacle ships u/1 -> Predict obstacle trajectories/10(SBMPC_obstacle_ships_u)
  SBMPC obstacle ships v/1 -> Predict obstacle trajectories/11(SBMPC_obstacle_ships_v)
  Predict obstacle trajectories/1(normal obstacle_ships_x_predicted) -> normal obstacle_ships_x_predicted/1
  Predict obstacle trajectories/2("normal obstacle_ships_y_predicted ") -> "normal obstacle_ships_y_predicted "/1
  Predict obstacle trajectories/3(obs_x_predicted) -> Calculate control behaviors/2(obstacle_ships_x_predicted)
  Predict obstacle trajectories/4(obs_y_predicted) -> Calculate control behaviors/3("obstacle_ships_y_predicted ")
  Predict obstacle trajectories/5(obs_psi) -> Calculate control behaviors/4(obstacle_ships_psi)
  Predict obstacle trajectories/6(obs_u) -> Calculate control behaviors/5(obstacle_ships_u)
  Predict obstacle trajectories/7(obs_v) -> Calculate control behaviors/6(obstacle_ships_v)

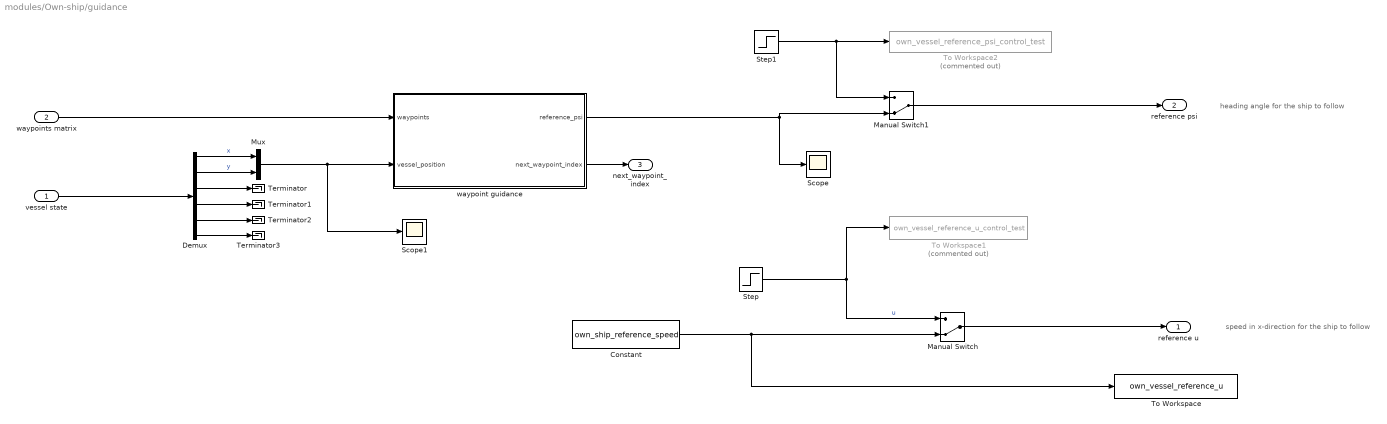
== system modules/Own-ship/guidance ==
  note: heading angle for the ship to follow
  note: speed in x-direction for the ship to follow
  vessel state : Inport
  "waypoints matrix " : Inport  Port=2
  Constant : Constant  Value=own_ship_reference_speed  SampleTime=tsamp
  Demux : Demux  Outputs=6
  Manual Switch : ManualSwitch  CurrentSetting=0
  Manual Switch1 : ManualSwitch  CurrentSetting=0
  Mux : Mux  Inputs=2
  Scope : Scope
  Scope1 : Scope
  Step : Step  Time=100  After=5  SampleTime=0
  Step1 : Step  Time=100  Before=eta_initial(3)  After=0*deg2rad  SampleTime=0
  Terminator{,1..3} (4 alike) : Terminator
  To Workspace : ToWorkspace  VariableName=own_vessel_reference_u  SampleTime=tsamp
  To Workspace1 : ToWorkspace  Commented=on  VariableName=own_vessel_reference_u_control_test  SampleTime=tsamp
      settings: Save2DSignal=2-D array (concatenate along first dimension)
  To Workspace2 : ToWorkspace  Commented=on  VariableName=own_vessel_reference_psi_control_test  SampleTime=tsamp
      settings: Save2DSignal=2-D array (concatenate along first dimension)
  waypoint guidance : MATLAB Function  TreatAsAtomicUnit=on
  reference u : Outport
  "reference psi " : Outport  Port=2
  next_waypoint_index : Outport  Port=3
  wires:
  Constant/1 -> To Workspace/1, Manual Switch/2
  "waypoints matrix "/1 -> waypoint guidance/1(waypoints)
  vessel state/1 -> Demux/1
  Step/1 -> To Workspace1/1, Manual Switch/1  "u"
  Step1/1 -> To Workspace2/1, Manual Switch1/1
  Manual Switch/1 -> reference u/1
  Demux/1 -> Mux/1  "x"
  Demux/2 -> Mux/2  "y"
  Manual Switch1/1 -> "reference psi "/1
  Demux/3 -> Terminator/1
  Demux/4 -> Terminator1/1
  Demux/5 -> Terminator2/1
  Demux/6 -> Terminator3/1
  waypoint guidance/1(reference_psi) -> Manual Switch1/2, Scope/1
  Mux/1 -> Scope1/1, waypoint guidance/2(vessel_position)
  waypoint guidance/2(next_waypoint_index) -> next_waypoint_index/1

== system modules/Own-ship/reference model nu ==
  reference u : Inport
  Demux : Demux  Outputs=6
  MATLAB Function : MATLAB Function  TreatAsAtomicUnit=on
  Mux : Mux  Inputs=3
  Scope2 : Scope
  Scope3 : Scope
  Terminator : Terminator
  Terminator1 : Terminator
  Terminator2 : Terminator
  To Workspace2 : ToWorkspace  VariableName=own_vessel_desired_u  SampleTime=tsamp
      settings: Save2DSignal=2-D array (concatenate along first dimension)
  desired_nu : Outport
  wires:
  reference u/1 -> MATLAB Function/1(reference_u)
  MATLAB Function/1(x_d_new) -> Demux/1
  Demux/1 -> Mux/1, To Workspace2/1  "desired_u"
  Demux/2 -> Scope2/1, Mux/2  "desired_v"
  Demux/3 -> Scope3/1, Mux/3  "desired_r"
  Mux/1 -> desired_nu/1
  Demux/4 -> Terminator/1
  Demux/5 -> Terminator1/1
  Demux/6 -> Terminator2/1

== system modules/Own-ship/reference model psi ==
  reference psi : Inport
  Demux : Demux  Outputs=9
  Scope : Scope
  Scope1 : Scope
  Scope2 : Scope
  Terminator{,1..5} (6 alike) : Terminator
  To Workspace : ToWorkspace  VariableName=own_vessel_reference_psi  SampleTime=tsamp
  To Workspace1 : ToWorkspace  VariableName=own_vessel_desired_psi  SampleTime=tsamp
  own ship reference model psi : MATLAB Function  TreatAsAtomicUnit=on
  desired psi : Outport
  wires:
  reference psi/1 -> own ship reference model psi/1(reference_psi), To Workspace/1
  own ship reference model psi/1(x_d_new) -> Demux/1
  Demux/3 -> To Workspace1/1, Scope/1, desired psi/1  "desired psi"
  Demux/1 -> Scope1/1  "desired x"
  Demux/2 -> Scope2/1  "desired y"
  Demux/4 -> Terminator/1
  Demux/5 -> Terminator1/1
  Demux/6 -> Terminator2/1
  Demux/7 -> Terminator3/1
  Demux/8 -> Terminator4/1
  Demux/9 -> Terminator5/1

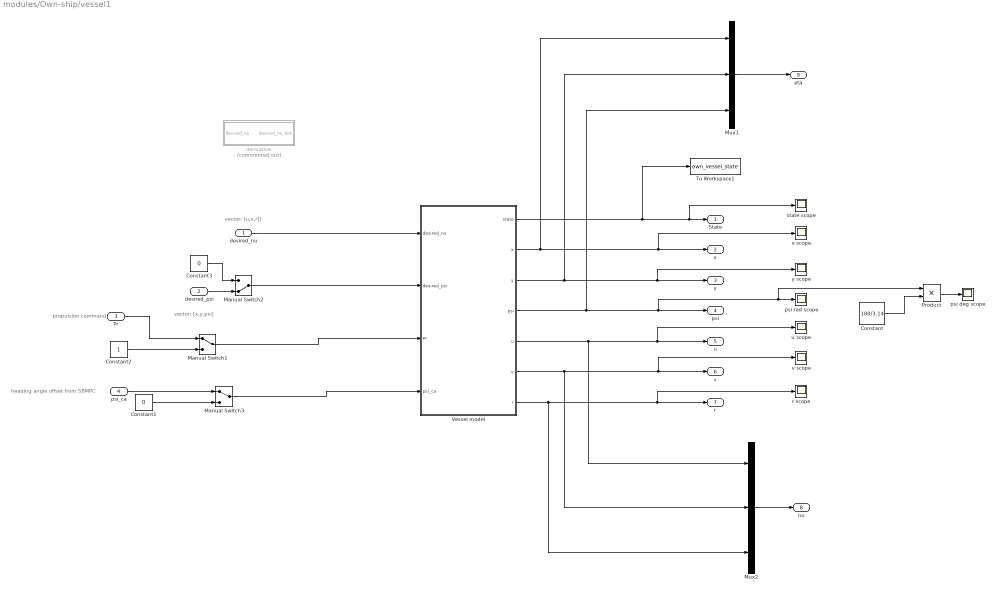
== system modules/Own-ship/vessel1 ==
  note: heading angle offset from SBMPC
  note: propulsion command
  note: vector: [x,y,psi]
  note: vector: [u,v,r]]
  desired_nu : Inport
  "desired_psi " : Inport  Port=2
  Pr : Inport  Port=3
  psi_ca : Inport  Port=4
  Constant : Constant  Value=180/3.14  SampleTime=time_step
  Constant1 : Constant  Value=0
  Constant2 : Constant
  Constant3 : Constant  Value=0
  Manual Switch1 : ManualSwitch
  Manual Switch2 : ManualSwitch  CurrentSetting=0
  Manual Switch3 : ManualSwitch
  Mux1 : Mux  Inputs=3
  Mux2 : Mux  Inputs=3
  Product : Product
  To Workspace1 : ToWorkspace  VariableName=own_vessel_state  SampleTime=tsamp
  Vessel model : Subsystem
  derivative : Subsystem  Commented=on
  psi deg scope : Scope
  psi rad scope : Scope
  r scope : Scope
  "state scope " : Scope
  u scope : Scope
  v scope : Scope
  "x scope " : Scope
  y scope : Scope
  "State " : Outport  PortDimensions=state_dimension
  x : Outport  Port=2  PortDimensions=1
  y : Outport  Port=3  PortDimensions=1
  psi : Outport  Port=4  PortDimensions=1
  u : Outport  Port=5  PortDimensions=1
  v : Outport  Port=6  PortDimensions=1
  r : Outport  Port=7  PortDimensions=1
  nu : Outport  Port=8
  eta : Outport  Port=9
  wires:
  Vessel model/1(state) -> To Workspace1/1, "state scope "/1, "State "/1
  Vessel model/5(u) -> Mux2/1, u/1, u scope/1
  Vessel model/6(v) -> Mux2/2, v/1, v scope/1
  Vessel model/3(y) -> Mux1/2, y/1, y scope/1
  Vessel model/2(x) -> Mux1/1, x/1, "x scope "/1
  Vessel model/7(r) -> Mux2/3, r/1, r scope/1
  Vessel model/4(psi) -> Mux1/3, psi/1, Product/1, psi rad scope/1
  Constant/1 -> Product/2
  Product/1 -> psi deg scope/1
  desired_nu/1 -> Vessel model/1(desired_nu)
  Manual Switch2/1 -> Vessel model/2(desired_psi)
  "desired_psi "/1 -> Manual Switch2/2
  Constant3/1 -> Manual Switch2/1
  Mux2/1 -> nu/1
  Mux1/1 -> eta/1
  Pr/1 -> Manual Switch1/1
  Manual Switch1/1 -> Vessel model/3(Pr)
  psi_ca/1 -> Manual Switch3/1
  Manual Switch3/1 -> Vessel model/4(psi_ca)
  Constant2/1 -> Manual Switch1/2
  Constant1/1 -> Manual Switch3/2

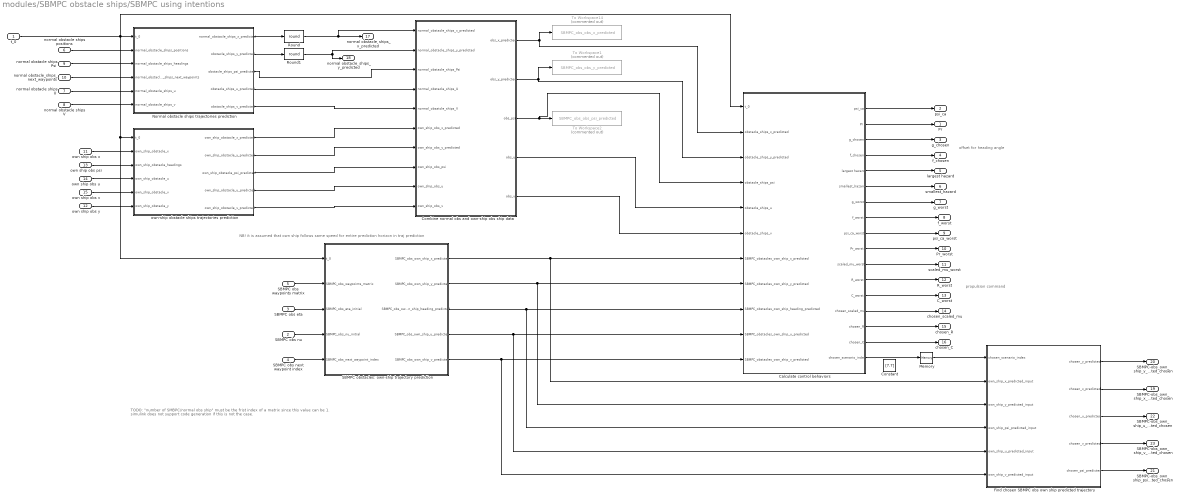
== system modules/SBMPC obstacle ships/SBMPC using intentions  ==
  note: TODO: "number of SMBPC/normal obs ship" must be the frist index of a matrix since this value can be 1. simulink
      | does not support code generation if this is not the case.
  note: propulsion command
  note: offset for heading angle
  note: NB! it is assumed that own ship follows same speed for entire prediction horizon in traj prediction
  t_0 : Inport
  SBMPC obs nu : Inport  Port=2
  SBMPC obs eta : Inport  Port=3
  SBMPC obs next waypoint index : Inport  Port=4
  "SBMPC obs waypoints matrix " : Inport  Port=5
  normal obstacle ships positions : Inport  Port=6
  normal obstacle ships U : Inport  Port=7
  normal obstacle ships V : Inport  Port=8
  normal obstacle ships Psi : Inport  Port=9
  normal obstacle_ships_next_waypoints : Inport  Port=10
  "own ship obs x " : Inport  Port=11  SampleTime=time_step
  "own ship obs y " : Inport  Port=12  SampleTime=time_step
  "own ship obs psi " : Inport  Port=13
  "own ship obs u " : Inport  Port=14
  "own ship obs v " : Inport  Port=15
  Calculate control behaviors : Subsystem
  "Combine normal obs and own-ship obs ship data " : MATLAB Function  TreatAsAtomicUnit=on
  Constant : Constant  Value=[7,7]  VectorParams1D=off
  Find chosen SBMPC obs own ship predicted trajectory : MATLAB Function  TreatAsAtomicUnit=on
  Memory : Memory  X0=7
  Normal obstacle ships trajectories prediction : Subsystem
  Round : Rounding  Operator=round
  Round1 : Rounding  Operator=round
  SBMPC obstacles: own-ship trajectory prediction : Subsystem
  To Workspace1 : ToWorkspace  Commented=on  VariableName=SBMPC_obs_obs_y_predicted  SaveFormat=Structure With Time  SampleTime=tsamp
      settings: Save2DSignal=2-D array (concatenate along first dimension)
  To Workspace14 : ToWorkspace  Commented=on  VariableName=SBMPC_obs_obs_x_predicted  SaveFormat=Structure With Time  SampleTime=tsamp
      settings: Save2DSignal=2-D array (concatenate along first dimension)
  To Workspace2 : ToWorkspace  Commented=on  VariableName=SBMPC_obs_obs_psi_predicted  SaveFormat=Structure With Time  SampleTime=tsamp
      settings: Save2DSignal=2-D array (concatenate along first dimension)
  own-ship obstacle ships trajectories prediction : Subsystem
  Pr : Outport
  psi_ca : Outport  Port=2
  "g_chosen " : Outport  Port=3  SampleTime=time_step
  f_chosen : Outport  Port=4  SampleTime=time_step
  largest hazard : Outport  Port=5  SampleTime=time_step
  smallest_hazard : Outport  Port=6  SampleTime=time_step
  "g_worst " : Outport  Port=7  SampleTime=time_step
  f_worst : Outport  Port=8  SampleTime=time_step
  psi_ca_worst : Outport  Port=9  SampleTime=time_step
  Pr_worst : Outport  Port=10  SampleTime=time_step
  scaled_mu_worst : Outport  Port=11  SampleTime=time_step
  R_worst : Outport  Port=12  SampleTime=time_step
  C_worst : Outport  Port=13  SampleTime=time_step
  chosen_scaled_mu : Outport  Port=14  SampleTime=time_step
  chosen_R : Outport  Port=15  SampleTime=time_step
  chosen_C : Outport  Port=16  SampleTime=time_step
  normal obstacle_ships_x_predicted : Outport  Port=17  SampleTime=time_step
  "normal obstacle_ships_y_predicted " : Outport  Port=18  SampleTime=time_step
  SBMPC-obs_own_ship_x_predicted_chosen : Outport  Port=19  SampleTime=time_step
  SBMPC-obs_own_ship_y_predicted_chosen : Outport  Port=20  SampleTime=time_step
  SBMPC-obs_own_ship_psi_predicted_chosen : Outport  Port=21  SampleTime=time_step
  SBMPC-obs_own_ship_u_predicted_chosen : Outport  Port=22  SampleTime=time_step
  SBMPC-obs_own_ship_v_predicted_chosen : Outport  Port=23  SampleTime=time_step
  wires:
  "SBMPC obs waypoints matrix "/1 -> SBMPC obstacles: own-ship trajectory prediction/2(SBMPC_obs_waypoints_matrix)
  SBMPC obs eta/1 -> SBMPC obstacles: own-ship trajectory prediction/3("SBMPC_obs_eta_initial ")
  SBMPC obs nu/1 -> SBMPC obstacles: own-ship trajectory prediction/4(SBMPC_obs_nu_initial)
  SBMPC obs next waypoint index/1 -> SBMPC obstacles: own-ship trajectory prediction/5(SBMPC_obs_next_waypoint_index)
  t_0/1 -> own-ship obstacle ships trajectories prediction/1(t_0), SBMPC obstacles: own-ship trajectory prediction/1(t_0), Calculate control behaviors/1(t_0), Normal obstacle ships trajectories prediction/1(t_0)
  normal obstacle ships positions/1 -> Normal obstacle ships trajectories prediction/2(normal_obstacle_ships_positions)
  normal obstacle ships Psi/1 -> Normal obstacle ships trajectories prediction/3(normal_obstacle_ships_headings)
  SBMPC obstacles: own-ship trajectory prediction/5("SBMPC_obs_own_ship_v_predicted ") -> Find chosen SBMPC obs own ship predicted trajectory/6(own_ship_v_predicted_input), Calculate control behaviors/11("SBMPC_obstacles_own_ship_v_predicted ")
  SBMPC obstacles: own-ship trajectory prediction/3(SBMPC_obs_own_ship_heading_predicted) -> Calculate control behaviors/9("SBMPC_obstacles_own_ship_heading_predicted "), Find chosen SBMPC obs own ship predicted trajectory/4(own_ship_psi_predicted_input)
  Calculate control behaviors/2(Pr) -> Pr/1
  Calculate control behaviors/1(psi_ca) -> psi_ca/1
  normal obstacle_ships_next_waypoints/1 -> Normal obstacle ships trajectories prediction/4(normal_obstacle_ships_next_waypoints)
  Calculate control behaviors/16(chosen_C) -> chosen_C/1
  Calculate control behaviors/15(chosen_R) -> chosen_R/1
  Calculate control behaviors/14(chosen_scaled_mu) -> chosen_scaled_mu/1
  Calculate control behaviors/13(C_worst) -> C_worst/1
  Calculate control behaviors/12(R_worst) -> R_worst/1
  Calculate control behaviors/11(scaled_mu_worst) -> scaled_mu_worst/1
  Calculate control behaviors/10(Pr_worst) -> Pr_worst/1
  Calculate control behaviors/9(psi_ca_worst) -> psi_ca_worst/1
  Calculate control behaviors/8(f_worst) -> f_worst/1
  Calculate control behaviors/7("g_worst ") -> "g_worst "/1
  Calculate control behaviors/6(smallest_hazard) -> smallest_hazard/1
  Calculate control behaviors/5(largest hazard) -> largest hazard/1
  Calculate control behaviors/4(f_chosen) -> f_chosen/1
  Calculate control behaviors/3("g_chosen ") -> "g_chosen "/1
  "Combine normal obs and own-ship obs ship data "/5(obs_v) -> Calculate control behaviors/6(obstacle_ships_v)
  "Combine normal obs and own-ship obs ship data "/4(obs_u) -> Calculate control behaviors/5(obstacle_ships_u)
  "Combine normal obs and own-ship obs ship data "/3(obs_psi) -> Calculate control behaviors/4(obstacle_ships_psi), To Workspace2/1
  "Combine normal obs and own-ship obs ship data "/2(obs_y_predicted) -> Calculate control behaviors/3("obstacle_ships_y_predicted "), To Workspace1/1
  "Combine normal obs and own-ship obs ship data "/1(obs_x_predicted) -> Calculate control behaviors/2(obstacle_ships_x_predicted), To Workspace14/1
  SBMPC obstacles: own-ship trajectory prediction/1(SBMPC_obs_own_ship_x_predicted) -> Find chosen SBMPC obs own ship predicted trajectory/2(own_ship_x_predicted_input), Calculate control behaviors/7(SBMPC_obstacles_own_ship_x_predicted)
  SBMPC obstacles: own-ship trajectory prediction/2(SBMPC_obs_own_ship_y_predicted) -> Find chosen SBMPC obs own ship predicted trajectory/3(own_ship_y_predicted_input), Calculate control behaviors/8(SBMPC_obstacles_own_ship_y_predicted)
  SBMPC obstacles: own-ship trajectory prediction/4(SBMPC_obs_own_ship_u_predicted) -> Find chosen SBMPC obs own ship predicted trajectory/5(own_ship_u_predicted_input), Calculate control behaviors/10(SBMPC_obstacles_own_ship_u_predicted)
  Memory/1 -> Find chosen SBMPC obs own ship predicted trajectory/1(chosen_scenario_index)
  Find chosen SBMPC obs own ship predicted trajectory/1(chosen_y_predicted) -> SBMPC-obs_own_ship_y_predicted_chosen/1
  Find chosen SBMPC obs own ship predicted trajectory/2(chosen_x_predicted) -> SBMPC-obs_own_ship_x_predicted_chosen/1
  Find chosen SBMPC obs own ship predicted trajectory/3(chosen_u_predicted) -> SBMPC-obs_own_ship_u_predicted_chosen/1
  Find chosen SBMPC obs own ship predicted trajectory/4(chosen_v_predicted) -> SBMPC-obs_own_ship_v_predicted_chosen/1
  Find chosen SBMPC obs own ship predicted trajectory/5(chosen_psi_predicted) -> SBMPC-obs_own_ship_psi_predicted_chosen/1
  Normal obstacle ships trajectories prediction/2(obstacle_ships_y_predicted) -> Round1/1
  Normal obstacle ships trajectories prediction/3(obstacle_ships_psi_predicted) -> "Combine normal obs and own-ship obs ship data "/3(normal_obstacle_ships_Psi)
  Normal obstacle ships trajectories prediction/4(obstacle_ships_u_predicted) -> "Combine normal obs and own-ship obs ship data "/4(normal_obstacle_ships_U)
  Normal obstacle ships trajectories prediction/5(obstacle_ships_v_predicted) -> "Combine normal obs and own-ship obs ship data "/5(normal_obsatcle_ships_V)
  Normal obstacle ships trajectories prediction/1(normal_obstacle_ships_x_predicted) -> Round/1
  normal obstacle ships U/1 -> Normal obstacle ships trajectories prediction/5(normal_obstacle_ships_u)
  normal obstacle ships V/1 -> Normal obstacle ships trajectories prediction/6(normal_obstacle_ships_v)
  Calculate control behaviors/17(chosen_scenario_index) -> Memory/1
  own-ship obstacle ships trajectories prediction/1(own_ship_obstacle_x_predicted) -> "Combine normal obs and own-ship obs ship data "/6(own_ship_obs_x_predicted)
  own-ship obstacle ships trajectories prediction/2(own_ship_obstacle_y_predicted) -> "Combine normal obs and own-ship obs ship data "/7(own_ship_obs_y_predicted)
  own-ship obstacle ships trajectories prediction/3(own_ship_obstacle_psi_predicted) -> "Combine normal obs and own-ship obs ship data "/8(own_ship_obs_psi)
  own-ship obstacle ships trajectories prediction/4(own_ship_obstacle_u_predicted) -> "Combine normal obs and own-ship obs ship data "/9(own_ship_obs_u)
  own-ship obstacle ships trajectories prediction/5(own_ship_obstacle_v_predicted) -> "Combine normal obs and own-ship obs ship data "/10(own_ship_obs_v)
  "own ship obs x "/1 -> own-ship obstacle ships trajectories prediction/2(own_ship_obstacle_x)
  "own ship obs psi "/1 -> own-ship obstacle ships trajectories prediction/3(own_ship_obstacle_headings)
  "own ship obs u "/1 -> own-ship obstacle ships trajectories prediction/4(own_ship_obstacle_u)
  "own ship obs y "/1 -> own-ship obstacle ships trajectories prediction/6(own_ship_obstacle_y)
  "own ship obs v "/1 -> own-ship obstacle ships trajectories prediction/5(own_ship_obstacle_v)
  Round/1 -> normal obstacle_ships_x_predicted/1, "Combine normal obs and own-ship obs ship data "/1(normal_obstacle_ships_x_predicted)
  Round1/1 -> "normal obstacle_ships_y_predicted "/1, "Combine normal obs and own-ship obs ship data "/2(normal_obstacle_ships_y_predicted)

== system modules/SBMPC obstacle ships/guidance  ==
  state matrix : Inport
  "waypoints matrix " : Inport  Port=2
  SBMPC obstacle waypoint guidance : MATLAB Function  TreatAsAtomicUnit=on
  SBMPC reference u vector : MATLAB Function  TreatAsAtomicUnit=on
  Scope : Scope
  Scope1 : Scope
  Scope2 : Scope
  "reference psi " : Outport
  reference u vector : Outport  Port=2
  "next_waypoints_indexes " : Outport  Port=3
  wires:
  "waypoints matrix "/1 -> SBMPC obstacle waypoint guidance/1(SBMPC_obstacle_waypoints)
  state matrix/1 -> SBMPC obstacle waypoint guidance/2(state_matrix)
  SBMPC obstacle waypoint guidance/1(reference_psi_vector) -> "reference psi "/1, Scope/1
  SBMPC reference u vector/1(u_vector) -> Scope2/1, reference u vector/1
  SBMPC obstacle waypoint guidance/2(next_waypoints_indexes) -> SBMPC reference u vector/1(next_waypoints_indexes), Scope1/1, "next_waypoints_indexes "/1

== system modules/SBMPC obstacle ships/reference model for psi ==
  note: row vector
  note: row vector
  reference psi vector : Inport
  "SBMPC psi reference model " : MATLAB Function  TreatAsAtomicUnit=on
  Scope3 : Scope  NumInputPorts=2
  To Workspace : ToWorkspace  VariableName=SBMPC_obstacle_ships_reference_psi_vector  SampleTime=tsamp
      settings: Save2DSignal=2-D array (concatenate along first dimension)
  To Workspace1 : ToWorkspace  VariableName=SBMPC_obstacle_ships_desired_psi_vector  SampleTime=tsamp
      settings: Save2DSignal=2-D array (concatenate along first dimension)
  "desired psi vector " : Outport
  wires:
  "SBMPC psi reference model "/1(desired_psi_vector) -> Scope3/1, To Workspace1/1, "desired psi vector "/1
  reference psi vector/1 -> Scope3/2, To Workspace/1, "SBMPC psi reference model "/1(reference_psi_vector)

== system modules/SBMPC obstacle ships/reference model for u ==
  note: row vector
  note: row vector
  "reference u vector " : Inport
  SBMPC obstacle ships reference model u : MATLAB Function  TreatAsAtomicUnit=on
  To Workspace : ToWorkspace  VariableName=SBMPC_obstacle_ships_reference_u_vector  SampleTime=tsamp
      settings: Save2DSignal=2-D array (concatenate along first dimension)
  To Workspace1 : ToWorkspace  VariableName=SBMPC_obstacle_ships_desired_u_vector  SampleTime=tsamp
      settings: Save2DSignal=2-D array (concatenate along first dimension)
  desired_u_vector : Outport
  wires:
  "reference u vector "/1 -> To Workspace/1, SBMPC obstacle ships reference model u/1(reference_u_vetor)
  SBMPC obstacle ships reference model u/1(desired_u_vector) -> To Workspace1/1, desired_u_vector/1
